simulink model "P_3"  (R2019a)
settings: Solver=VariableStepAuto  StartTime=0.0  StopTime=10.0  RelTol=1e-3
settings Model: Creator=john  LastModifiedBy=john

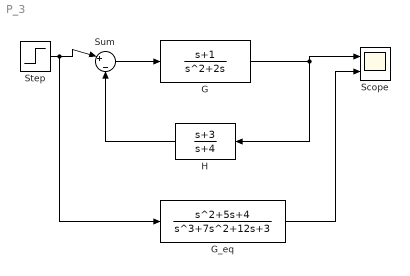
== system P_3 ==
  G : TransferFcn  Numerator=[1 1]  Denominator=[1 2 0]
  G_eq : TransferFcn  Numerator=[1 5 4]  Denominator=[1 7 12 3]
  H : TransferFcn  Numerator=[1 3]  Denominator=[1 4]
  Scope : Scope  NumInputPorts=2
  Step : Step  SampleTime=0
  Sum : Sum  Inputs=|+|-
  wires:
  H/1 -> Sum/2
  Sum/1 -> G/1
  G/1 -> Scope/1, H/1
  G_eq/1 -> Scope/2
  Step/1 -> G_eq/1, Sum/1
